simulink model "Day18"  (R2024b)
settings: Solver=VariableStepAuto  StartTime=0.0  StopTime=10.0  RelTol=1e-3
settings Model: Creator=jun_mac  LastModifiedBy=jun_mac

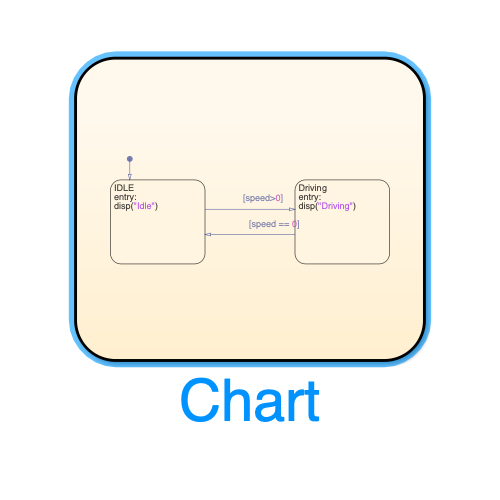
[thumbnail: Simulink's stored preview of the top-level diagram]
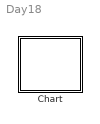
== system Day18 ==
  Chart : Stateflow chart  TreatAsAtomicUnit=on

== stateflow chart Day18/Chart ==
  state IDLE
    entry:
    disp("Idle")
  state Driving
    entry:
    disp("Driving")
  (default) -> IDLE
  IDLE -> Driving : true
  Driving -> IDLE : true
